simulink model "SMC"  (R2023a)
settings: Solver=VariableStepAuto  StartTime=0.0  StopTime=50  RelTol=1e-3
settings Model: Creator=30296  LastModifiedBy=30296

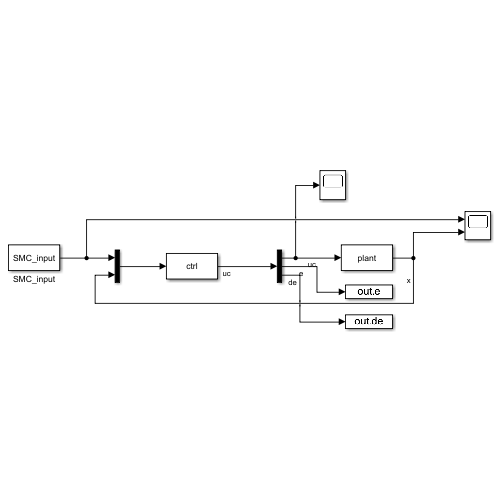
[thumbnail: Simulink's stored preview of the top-level diagram]
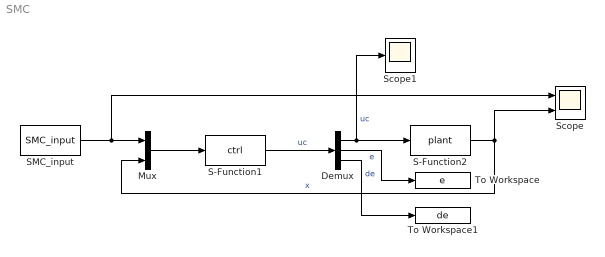
== system SMC ==
  Demux : Demux  Outputs=3
  Mux : Mux  Inputs=2
  S-Function1 : S-Function  FunctionName=ctrl  Parameters=pa  SFunctionDeploymentMode=off  EnableBusSupport=off
  S-Function2 : S-Function  FunctionName=plant  Parameters=pa  SFunctionDeploymentMode=off  EnableBusSupport=off
  SMC_input : S-Function  FunctionName=SMC_input  Parameters=pa  SFunctionDeploymentMode=off  EnableBusSupport=off
  Scope : Scope  NumInputPorts=2
  Scope1 : Scope
  To Workspace : ToWorkspace  VariableName=e  SampleTime=-1
  To Workspace1 : ToWorkspace  VariableName=de  SampleTime=-1
  wires:
  Mux/1 -> S-Function1/1
  SMC_input/1 -> Scope/1, Mux/1
  S-Function2/1 -> Mux/2, Scope/2  "x"
  S-Function1/1 -> Demux/1  "uc"
  Demux/1 -> Scope1/1, S-Function2/1  "uc"
  Demux/2 -> To Workspace/1  "e"
  Demux/3 -> To Workspace1/1  "de"
